simulink model "system_EKF_rendes"  (R2020b)
settings: Solver=VariableStepAuto  StartTime=0.0  StopTime=5  RelTol=1e-3
values from neighbouring files (symbols this model uses):
  e1_noise_std = 0.05    [system_EKF_rendes_ws.m]
  e2_noise_std = deg2rad(0.5)    [system_EKF_rendes_ws.m]
  P0 = eye(4) * 1000    [system_EKF_rendes_ws.m]
  Q = Q_e1 + Q_e2    [system_EKF_rendes_ws.m]
  R = diag([e1_noise_std^2, e2_noise_std^2])    [system_EKF_rendes_ws.m]
  T = 0.01    [ode_try.m]    (also in system_EKF_rendes_ws.m = 0.033)
  threshold = 1    [system_EKF_rendes_ws.m]
  vehicleParams = struct('Cf', Cf, 'Cr', Cr, 'lf', lf, 'lr', lr, 'm', m, 'Iz', Iz)    [system_EKF_rendes_ws.m]
  x0 = x_Prior    [ode_try.m]    (also in system_EKF_rendes_ws.m = zeros(4, 1))
settings Model: Creator=Lindenmaier  LastModifiedBy=Admin

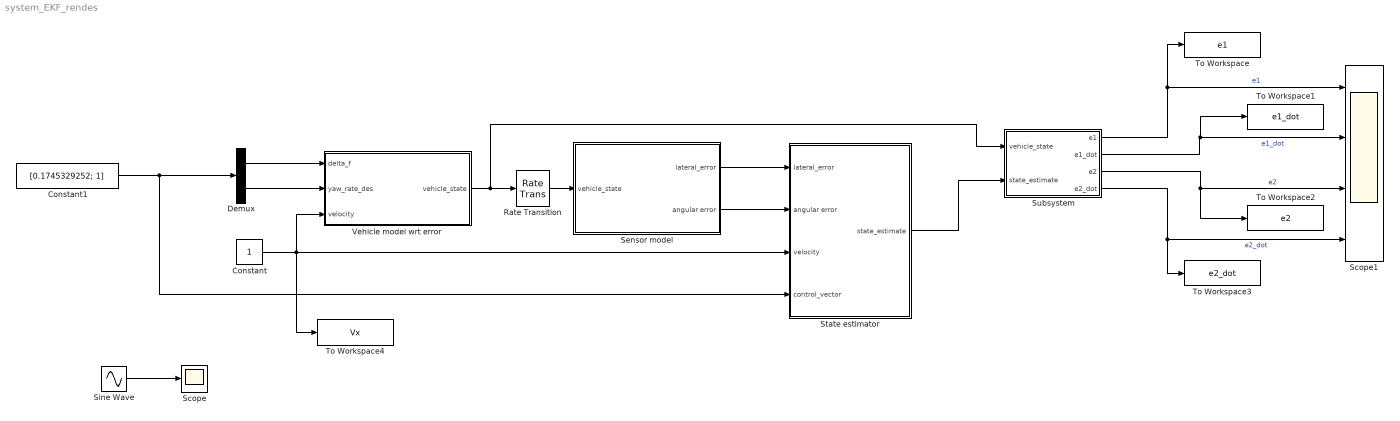
== system system_EKF_rendes ==
  Constant : Constant
  Constant1 : Constant  Value=[0.1745329252; 1]
  Demux : Demux  Outputs=2
  Rate Transition : RateTransition  OutPortSampleTime=T
  Scope : Scope
  Scope1 : Scope  NumInputPorts=4
  Sensor model : Subsystem
  Sine Wave : Sin  Amplitude=10  Frequency=0.5  SampleTime=T
  State estimator : Subsystem
  Subsystem : Subsystem
  To Workspace : ToWorkspace  VariableName=e1  SaveFormat=Timeseries  SampleTime=-1
  To Workspace1 : ToWorkspace  VariableName=e1_dot  SaveFormat=Timeseries  SampleTime=-1
  To Workspace2 : ToWorkspace  VariableName=e2  SaveFormat=Timeseries  SampleTime=-1
  To Workspace3 : ToWorkspace  VariableName=e2_dot  SaveFormat=Timeseries  SampleTime=-1
  To Workspace4 : ToWorkspace  VariableName=Vx  SaveFormat=Timeseries  SampleTime=-1
  Vehicle model wrt error : Subsystem
  wires:
  Vehicle model wrt error/1(vehicle_state) -> Subsystem/1(vehicle_state), Rate Transition/1
  Rate Transition/1 -> Sensor model/1(vehicle_state)
  Sensor model/1(lateral_error) -> State estimator/1(lateral_error)
  Sensor model/2(angular error) -> State estimator/2(angular error)
  Constant/1 -> To Workspace4/1, State estimator/3(velocity), Vehicle model wrt error/3(velocity)
  Constant1/1 -> State estimator/4(control_vector), Demux/1
  Demux/1 -> Vehicle model wrt error/1(delta_f)
  Demux/2 -> Vehicle model wrt error/2(yaw_rate_des)
  State estimator/1(state_estimate) -> Subsystem/2(state_estimate)
  Subsystem/1(e1) -> To Workspace/1, Scope1/1  "e1"
  Subsystem/2(e1_dot) -> To Workspace1/1, Scope1/2  "e1_dot"
  Subsystem/3(e2) -> To Workspace2/1, Scope1/3  "e2"
  Subsystem/4(e2_dot) -> To Workspace3/1, Scope1/4  "e2_dot"
  Sine Wave/1 -> Scope/1

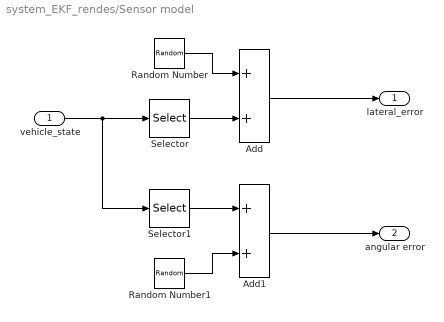
== system system_EKF_rendes/Sensor model ==
  vehicle_state : Inport
  Add : Sum
  Add1 : Sum
  Random Number : RandomNumber  Variance=e1_noise_std^2  SampleTime=T
  Random Number1 : RandomNumber  Variance=e2_noise_std^2  Seed=1  SampleTime=T
  Selector : Selector  InputPortWidth=4  IndexOptions=Index vector (dialog)  Indices=1  OutputSizes=1
  Selector1 : Selector  InputPortWidth=4  IndexOptions=Index vector (dialog)  Indices=3  OutputSizes=1
  lateral_error : Outport
  angular error : Outport  Port=2
  wires:
  vehicle_state/1 -> Selector1/1, Selector/1
  Selector/1 -> Add/2
  Random Number/1 -> Add/1
  Selector1/1 -> Add1/1
  Random Number1/1 -> Add1/2
  Add/1 -> lateral_error/1
  Add1/1 -> angular error/1

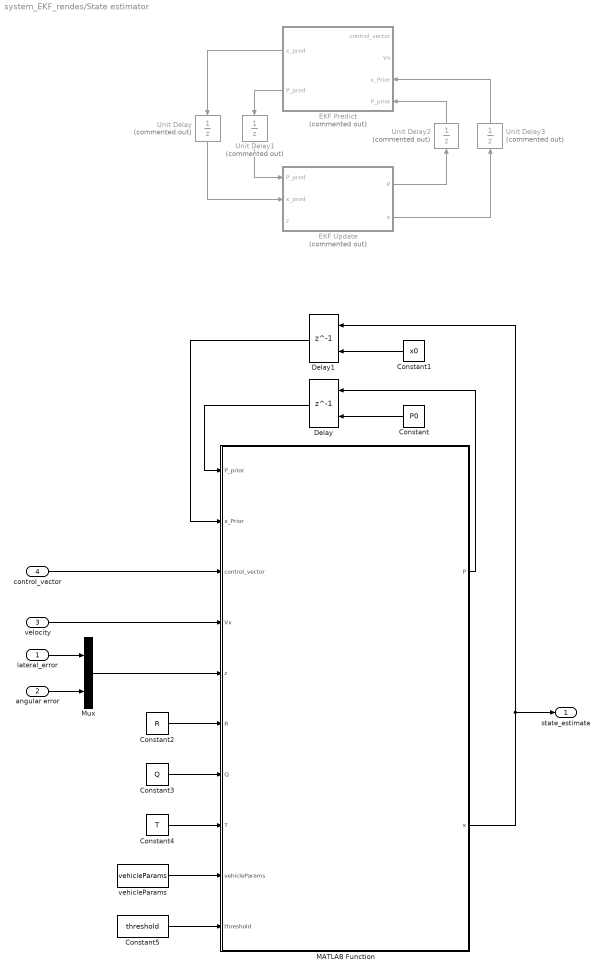
== system system_EKF_rendes/State estimator ==
  lateral_error : Inport
  angular error : Inport  Port=2
  velocity : Inport  Port=3
  control_vector : Inport  Port=4
  Constant : Constant  Value=P0
  Constant1 : Constant  Value=x0
  Constant2 : Constant  Value=R
  Constant3 : Constant  Value=Q
  Constant4 : Constant  Value=T
  Constant5 : Constant  Value=threshold
  Delay : Delay  DelayLength=1  InitialConditionSource=Input port
      settings: InputPortMap=u0,p4
  Delay1 : Delay  DelayLength=1  InitialConditionSource=Input port
      settings: InputPortMap=u0,p4
  EKF Predict : MATLAB Function  Commented=on  TreatAsAtomicUnit=on
  EKF Update : MATLAB Function  Commented=on  TreatAsAtomicUnit=on
  MATLAB Function : MATLAB Function  TreatAsAtomicUnit=on
  Mux : Mux  Inputs=2
  Unit Delay{,1..3} (4 alike) : UnitDelay  Commented=on  SampleTime=T  HasFrameUpgradeWarning=on
  vehicleParams : Constant  Value=vehicleParams  OutDataTypeStr=Bus: vehicleParamsBus
  state_estimate : Outport
  wires:
  lateral_error/1 -> Mux/1
  angular error/1 -> Mux/2
  EKF Update/2(x) -> Unit Delay3/1
  EKF Predict/1(x_pred) -> Unit Delay/1
  Unit Delay/1 -> EKF Update/2(x_pred)
  EKF Predict/2(P_pred) -> Unit Delay1/1
  Unit Delay1/1 -> EKF Update/1(P_pred)
  EKF Update/1(P) -> Unit Delay2/1
  Unit Delay2/1 -> EKF Predict/4(P_prior)
  Unit Delay3/1 -> EKF Predict/3(x_Prior)
  MATLAB Function/2(x) -> Delay1/1, state_estimate/1
  Mux/1 -> MATLAB Function/5(z)
  velocity/1 -> MATLAB Function/4(Vx)
  control_vector/1 -> MATLAB Function/3(control_vector)
  MATLAB Function/1(P) -> Delay/1
  Delay/1 -> MATLAB Function/1(P_prior)
  Delay1/1 -> MATLAB Function/2(x_Prior)
  Constant/1 -> Delay/2
  Constant1/1 -> Delay1/2
  Constant2/1 -> MATLAB Function/6(R)
  Constant3/1 -> MATLAB Function/7(Q)
  vehicleParams/1 -> MATLAB Function/9(vehicleParams)
  Constant4/1 -> MATLAB Function/8(T)
  Constant5/1 -> MATLAB Function/10(threshold)

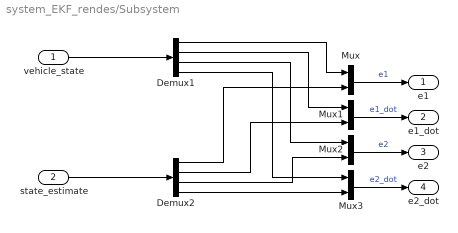
== system system_EKF_rendes/Subsystem ==
  vehicle_state : Inport
  state_estimate : Inport  Port=2
  Demux1 : Demux
  Demux2 : Demux
  Mux{,1..3} (4 alike) : Mux  Inputs=2
  e1 : Outport
  e1_dot : Outport  Port=2
  e2 : Outport  Port=3
  e2_dot : Outport  Port=4
  wires:
  Mux3/1 -> e2_dot/1  "e2_dot"
  Demux2/3 -> Mux2/2
  Demux1/1 -> Mux/1
  Demux2/1 -> Mux/2
  Demux2/2 -> Mux1/2
  Mux/1 -> e1/1  "e1"
  Demux1/2 -> Mux1/1
  Demux1/3 -> Mux2/1
  Demux1/4 -> Mux3/1
  Demux2/4 -> Mux3/2
  vehicle_state/1 -> Demux1/1
  state_estimate/1 -> Demux2/1
  Mux1/1 -> e1_dot/1  "e1_dot"
  Mux2/1 -> e2/1  "e2"

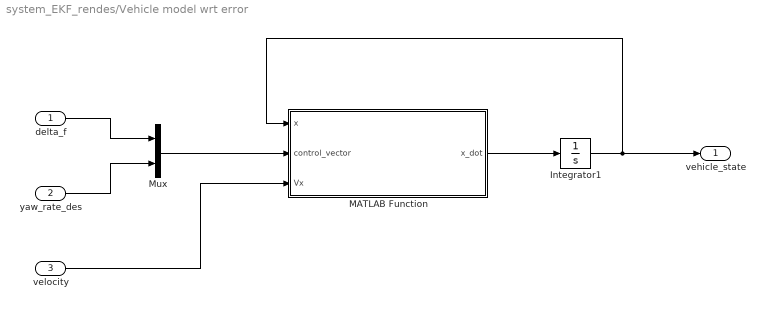
== system system_EKF_rendes/Vehicle model wrt error ==
  delta_f : Inport
  yaw_rate_des : Inport  Port=2
  velocity : Inport  Port=3
  Integrator1 : Integrator
  MATLAB Function : MATLAB Function  TreatAsAtomicUnit=on
  Mux : Mux  Inputs=2
  vehicle_state : Outport
  wires:
  Integrator1/1 -> MATLAB Function/1(x), vehicle_state/1
  yaw_rate_des/1 -> Mux/2
  delta_f/1 -> Mux/1
  MATLAB Function/1(x_dot) -> Integrator1/1
  Mux/1 -> MATLAB Function/2(control_vector)
  velocity/1 -> MATLAB Function/3(Vx)

== matlab function system_EKF_rendes/State estimator/EKF Predict ==
  data: control_vector input; Vx input; x_Prior input; x_pred output; P_pred output; P_prior input
function [x_pred, P_pred] = ekfPredict(control_vector, Vx, x_Prior, P_prior)

    % Parameters
    Cf=80000;
    Cr=80000;
    lf=1.4;
    lr=1.8;
    m=1500;
    Iz=1200;
    
    % Sampling period
    T = 0.1;

    % State-space model elements
    P1 = -((2*Cf + 2*Cr)/(m * Vx));
    P2 = (2*Cf + 2*Cr) / m;
    P3 = (-2*Cf * lf + 2*Cr * lr) / (m * Vx);
    P4 = -((2*Cf * lf - 2*Cr * lr) / (Iz * Vx));
    P5 = (2*Cf * lf - 2*Cr * lr) / Iz;
    P6 = -((2*Cf * lf^2 + 2*Cr * lr^2) / (Iz * Vx));
    P7 = (2*Cf) / m;
    P8 = -((2*Cf * lf - 2*Cr * lr) / (m * Vx)) - Vx;
    P9 = (2*Cf * lf) / Iz;
    P10 = -(2*Cf * lf^2 + 2*Cr * lr^2) / (Iz * Vx);

    % Continuous-time state-space matrices
    Ac = [0 1 0 0;
          0 P1 P2 P3;
          0 0 0 1;
          0 P4 P5 P6];
      
    Bc = [0 0;
          P7 P8;
          0 0;
          P9 P10];

    % Nonlinear state transition function
    F = Ac*x_Prior + Bc*control_vector;

    % Calculate Jacobian matrix of F with respect to x
    Jacobian_F = [0 1 0 0;
                  0 P1 P2 P3;
                  0 0 0 1;
                  0 P4 P5 P6];
    
    % Process noise covariance
    Q = eye(4) * 0.1; % Adjust as necessary
    I = eye(4); % Identity matrix

    % Time-update (prediction) step
    x_pred = x_Prior + T * F;
    P_pred = (I + T * Jacobian_F) * P_prior * (I + T * Jacobian_F)' + T * Q;
    
end

== matlab function system_EKF_rendes/State estimator/EKF Update ==
  data: P output; P_pred input; x_pred input; z input; x output
function [P, x] = ekfUpdate(P_pred, x_pred, z)

    % Measurement function (example: measuring only position states)
    h = [x_pred(1); x_pred(3)];

    % Calculate Jacobian matrix of h with respect to state
    Jacobian_H = [ 1, 0, 0, 0;
                   0, 0, 1, 0];

    % Measurement residual
    y = z - h;

    % Jacobian of measurement function at x_pred
    H = Jacobian_H;

    % Measurement noise covariance matrix (constant)
    R = eye(2) * 0.1;  % Adjust as necessary for your application

    % Innovation covariance
    S = H * P_pred * H' + R;

    % Optimal Kalman gain
    K = P_pred * H' / S;

    % Updated state estimate
    x = x_pred + K * y;

    % Updated estimate covariance
    P = (eye(size(P_pred)) - K * H) * P_pred;

end

== matlab function system_EKF_rendes/Vehicle model wrt error/MATLAB Function ==
  data: x input; x_dot output; control_vector input; Vx input
function x_dot = countinous_model(x, control_vector, Vx)

    % Parameters
    Cf=80000;
    Cr=80000;
    lf=1.4;
    lr=1.8;
    m=1500;
    Iz=1200;

    % Elements
    P1 = -((2*Cf+2*Cr)/(m*Vx));
    P2 = (2*Cf+2*Cr)/m;
    P3 = (-2*Cf*lf+2*Cr*lr)/(m*Vx);
    P4 = -((2*Cf*lf-2*Cr*lr)/(Iz*Vx));
    P5 = (2*Cf*lf-2*Cr*lr)/Iz;
    P6 = -((2*Cf*lf^2+2*Cr*lr^2)/(Iz*Vx));
    P7 = (2*Cf)/m;
    P8 = -((2*Cf*lf-2*Cr*lr)/(m*Vx))-Vx;
    P9 = (2*Cf*lf)/Iz;
    P10 = -(2*Cf*lf^2+2*Cr*lr^2)/(Iz*Vx);

    % State space
    Ac=[0 1  0  0;
        0 P1 P2 P3;
        0 0  0  1;
        0 P4 P5 P6]; 

    Bc=[0  0;
        P7 P8;
        0  0;
        P9 P10];
                  
x_dot = Ac*x + Bc*control_vector;

== matlab function system_EKF_rendes/State estimator/MATLAB Function ==
  data: P_prior input; x_Prior input; control_vector input; P output; Vx input; z input; x output; R input; Q input; T input; vehicleParams input; threshold input
function [P, x] = EKF_predict_update(P_prior, x_Prior, control_vector, Vx, z, R, Q, T, vehicleParams, threshold)

    % Parameters
    Cf = vehicleParams.Cf;
    Cr = vehicleParams.Cr;
    lf = vehicleParams.lf;
    lr = vehicleParams.lr;
    m  = vehicleParams.m;
    Iz = vehicleParams.Iz;

    % State-space model elements
    P1 = -((2*Cf + 2*Cr)/(m * Vx));
    P2 = (2*Cf + 2*Cr) / m;
    P3 = (-2*Cf * lf + 2*Cr * lr) / (m * Vx);
    P4 = -((2*Cf * lf - 2*Cr * lr) / (Iz * Vx));
    P5 = (2*Cf * lf - 2*Cr * lr) / Iz;
    P6 = -((2*Cf * lf^2 + 2*Cr * lr^2) / (Iz * Vx));
    P7 = (2*Cf) / m;
    P8 = -((2*Cf * lf - 2*Cr * lr) / (m * Vx)) - Vx;
    P9 = (2*Cf * lf) / Iz;
    P10 = -(2*Cf * lf^2 + 2*Cr * lr^2) / (Iz * Vx);

    % Continuous-time state-space matrices
    Ac = [0 1 0 0;
          0 P1 P2 P3;
          0 0 0 1;
          0 P4 P5 P6];
      
    Bc = [0 0;
          P7 P8;
          0 0;
          P9 P10];

    I = eye(4); % Identity matrix

    % Nonlinear state transition function
%     if abs(Vx) < threshold
%         Ad = 
%         Bd = 
%     else
%         Ad = (I + Ac * T);
%         Bd = Bc * T;
%     end
    
    Ad = (I + Ac * T);
    Bd = Bc * T;
    
    % Calculate Jacobian matrix of f() with respect to x
    F = Ac;
     

    % Time-update (prediction) step
    x_pred = Ad * x_Prior + Bd * control_vector;
    P_pred = (I + T * F) * P_prior * (I + T * F)' + Q;
    
    
    %%%%%%%%%%%%%%%%%%%%%%
    % Update
    % Measurement function (example: measuring only position states)
    h_x = [x_pred(1); x_pred(3)];

    % Calculate Jacobian matrix of h with respect to state
    H = [ 1, 0, 0, 0;
          0, 0, 1, 0];

    % Measurement residual
    y = z - h_x;

    % Innovation covariance
    S = H * P_pred * H' + R;

    % Optimal Kalman gain
    K = P_pred * H' / S;

    % Updated state estimate
    x = x_pred + K * y;

    % Updated estimate covariance
    P = (eye(size(P_pred)) - K * H) * P_pred;


end
